simulink model "six_plus_six_AcmsteeringV09_main_2lflm"  (R2014a)
settings: Solver=FixedStepDiscrete  StartTime=0.0  StopTime=10.0  FixedStep=0.0005  RelTol=1e-3
InitFcn:
  | Veh_Par_wxt
undefined symbols (not defined in the file or in its folder): acc_spdctl, ag_thr, B, bra_em, bra_pre_gz2, bra_pre_gz34, bra_pre_yd, brakepre_dem_data, brakeTrq_dem_data, bratrq_max, ecucoder_acal, eff_tran, ESP_switch, G, guzhang_lf, guzhang_lm, guzhang_lr, guzhang_rf, guzhang_rm, guzhang_rr, kd1, kd2, ki1, ki2, kp1, kp2, L, myFIS, premax, Radius, RC_switch, s_opt_yi, s_opt_zhuan, s_opt_zhuan_add, s_opt_zhuan_table, spd_map_mot, spd_spdctl, speed_thr_park, TCS_switch, tras_ratio, trq_map_mot, trqmax_yd, trqmax_zx, trqmaxneg, v_gain, v_table, v_thr_park, zhidong_bianmazhi, zhidong_down, zhidong_up, zhidong_youmen, zhuanxiang_bianmazhi, zhuanxiang_down, zhuanxiang_up, zhuanxiang_youmen
libraries: simulink x980, ec5744lib x59, fuzblock x2
(part 8 of 25)

== system six_plus_six_AcmsteeringV09_main_2lflm/Data_input/MCU0_1/MCU0 ==
  input : Inport
  Enable : EnablePort
  Demux : Demux  Outputs=8
  MCU0_ControlMode_Ad : Sum
  MCU0_ControlMode_Convert : DataTypeConversion  OutDataTypeStr=uint32
  MCU0_ControlMode_F : Gain
  MCU0_ControlMode_L : simulink/Logic and Bit Operations/Bitwise Operator  logicop=AND  UseBitMask=on  BitMask=4  BitMaskRealWorld=Stored Integer
  MCU0_ControlMode_O : Constant  Value=0  OutDataTypeStr=single
  MCU0_ControlMode_S : ArithShift  BitShiftNumber=2
  MCU0_ControlMode_Sub : Subsystem
  MCU0_ControlMode_sat : Saturate  UpperLimit=1  LowerLimit=0
  MCU0_ControlModecv : DataTypeConversion
  MCU0_EmergShutDown_Ad : Sum
  MCU0_EmergShutDown_Convert : DataTypeConversion  OutDataTypeStr=uint32
  MCU0_EmergShutDown_F : Gain
  MCU0_EmergShutDown_L : simulink/Logic and Bit Operations/Bitwise Operator  logicop=AND  UseBitMask=on  BitMask=128  BitMaskRealWorld=Stored Integer
  MCU0_EmergShutDown_O : Constant  Value=0  OutDataTypeStr=single
  MCU0_EmergShutDown_S : ArithShift  BitShiftNumber=7
  MCU0_EmergShutDown_Sub : Subsystem
  MCU0_EmergShutDown_sat : Saturate  UpperLimit=1  LowerLimit=0
  MCU0_EmergShutDowncv : DataTypeConversion
  MCU0_GearStatus_Ad : Sum
  MCU0_GearStatus_Convert : DataTypeConversion  OutDataTypeStr=uint32
  MCU0_GearStatus_F : Gain
  MCU0_GearStatus_L : simulink/Logic and Bit Operations/Bitwise Operator  logicop=AND  UseBitMask=on  BitMask=24  BitMaskRealWorld=Stored Integer
  MCU0_GearStatus_O : Constant  Value=0  OutDataTypeStr=single
  MCU0_GearStatus_S : ArithShift  BitShiftNumber=3
  MCU0_GearStatus_Sub : Subsystem
  MCU0_GearStatus_sat : Saturate  UpperLimit=3  LowerLimit=0
  MCU0_GearStatuscv : DataTypeConversion
  MCU0_HighVol_Ad : Sum
  MCU0_HighVol_Convert : DataTypeConversion  OutDataTypeStr=uint32
  MCU0_HighVol_F : Gain
  MCU0_HighVol_L : simulink/Logic and Bit Operations/Bitwise Operator  logicop=AND  UseBitMask=on  BitMask=32  BitMaskRealWorld=Stored Integer
  MCU0_HighVol_O : Constant  Value=0  OutDataTypeStr=single
  MCU0_HighVol_S : ArithShift  BitShiftNumber=5
  MCU0_HighVol_Sub : Subsystem
  MCU0_HighVol_sat : Saturate  UpperLimit=1  LowerLimit=0
  MCU0_HighVolcv : DataTypeConversion
  MCU0_LiftCnt_Ad : Sum
  MCU0_LiftCnt_Convert : DataTypeConversion  OutDataTypeStr=uint32
  MCU0_LiftCnt_F : Gain
  MCU0_LiftCnt_L : simulink/Logic and Bit Operations/Bitwise Operator  logicop=AND  UseBitMask=on  BitMask=255  BitMaskRealWorld=Stored Integer
  MCU0_LiftCnt_O : Constant  Value=0  OutDataTypeStr=single
  MCU0_LiftCnt_S : ArithShift
  MCU0_LiftCnt_Sub : Subsystem
  MCU0_LiftCnt_sat : Saturate  UpperLimit=255  LowerLimit=0
  MCU0_LiftCntcv : DataTypeConversion
  MCU0_ShutDowAllow_Ad : Sum
  MCU0_ShutDowAllow_Convert : DataTypeConversion  OutDataTypeStr=uint32
  MCU0_ShutDowAllow_F : Gain
  MCU0_ShutDowAllow_L : simulink/Logic and Bit Operations/Bitwise Operator  logicop=AND  UseBitMask=on  BitMask=64  BitMaskRealWorld=Stored Integer
  MCU0_ShutDowAllow_O : Constant  Value=0  OutDataTypeStr=single
  MCU0_ShutDowAllow_S : ArithShift  BitShiftNumber=6
  MCU0_ShutDowAllow_Sub : Subsystem
  MCU0_ShutDowAllow_sat : Saturate  UpperLimit=1  LowerLimit=0
  MCU0_ShutDowAllowcv : DataTypeConversion
  MCU0_SpeedFdk_Ad : Sum
  MCU0_SpeedFdk_Convert : DataTypeConversion  OutDataTypeStr=uint32
  MCU0_SpeedFdk_F : Gain
  MCU0_SpeedFdk_L : simulink/Logic and Bit Operations/Bitwise Operator  logicop=AND  UseBitMask=on  BitMask=65535  BitMaskRealWorld=Stored Integer
  MCU0_SpeedFdk_O : Constant  Value=-10000  OutDataTypeStr=single
  MCU0_SpeedFdk_S : ArithShift
  MCU0_SpeedFdk_Sub : Subsystem
  MCU0_SpeedFdk_sat : Saturate  UpperLimit=10000  LowerLimit=-10000
  MCU0_SpeedFdkcv : DataTypeConversion
  MCU0_SpeedFdkinput2_Ad : Sum
  MCU0_SpeedFdkinput2_C : Constant  Value=256
  MCU0_SpeedFdkinput2_P : Product
  MCU0_TorqueFdk_Ad : Sum
  MCU0_TorqueFdk_Convert : DataTypeConversion  OutDataTypeStr=uint32
  MCU0_TorqueFdk_F : Gain  Gain=0.1
  MCU0_TorqueFdk_L : simulink/Logic and Bit Operations/Bitwise Operator  logicop=AND  UseBitMask=on  BitMask=65535  BitMaskRealWorld=Stored Integer
  MCU0_TorqueFdk_O : Constant  Value=-1000  OutDataTypeStr=single
  MCU0_TorqueFdk_S : ArithShift
  MCU0_TorqueFdk_Sub : Subsystem
  MCU0_TorqueFdk_sat : Saturate  UpperLimit=1000  LowerLimit=-1000
  MCU0_TorqueFdkcv : DataTypeConversion
  MCU0_TorqueFdkinput4_Ad : Sum
  MCU0_TorqueFdkinput4_C : Constant  Value=256
  MCU0_TorqueFdkinput4_P : Product
  MCU0_TorqueMax_Ad : Sum
  MCU0_TorqueMax_Convert : DataTypeConversion  OutDataTypeStr=uint32
  MCU0_TorqueMax_F : Gain  Gain=0.1
  MCU0_TorqueMax_L : simulink/Logic and Bit Operations/Bitwise Operator  logicop=AND  UseBitMask=on  BitMask=65535  BitMaskRealWorld=Stored Integer
  MCU0_TorqueMax_O : Constant  Value=-1000  OutDataTypeStr=single
  MCU0_TorqueMax_S : ArithShift
  MCU0_TorqueMax_Sub : Subsystem
  MCU0_TorqueMax_sat : Saturate  UpperLimit=1000  LowerLimit=-1000
  MCU0_TorqueMaxcv : DataTypeConversion
  MCU0_TorqueMaxinput6_Ad : Sum
  MCU0_TorqueMaxinput6_C : Constant  Value=256
  MCU0_TorqueMaxinput6_P : Product
  MCU0_WorkStatus_Ad : Sum
  MCU0_WorkStatus_Convert : DataTypeConversion  OutDataTypeStr=uint32
  MCU0_WorkStatus_F : Gain
  MCU0_WorkStatus_L : simulink/Logic and Bit Operations/Bitwise Operator  logicop=AND  UseBitMask=on  BitMask=3  BitMaskRealWorld=Stored Integer
  MCU0_WorkStatus_O : Constant  Value=0  OutDataTypeStr=single
  MCU0_WorkStatus_S : ArithShift
  MCU0_WorkStatus_Sub : Subsystem
  MCU0_WorkStatus_sat : Saturate  UpperLimit=3  LowerLimit=0
  MCU0_WorkStatuscv : DataTypeConversion
  MCU0_TorqueMax_Out : Outport
  MCU0_EmergShutDown_Out : Outport  Port=2
  MCU0_ShutDowAllow_Out : Outport  Port=3
  MCU0_HighVol_Out : Outport  Port=4
  MCU0_LiftCnt_Out : Outport  Port=5
  MCU0_TorqueFdk_Out : Outport  Port=6
  MCU0_SpeedFdk_Out : Outport  Port=7
  MCU0_GearStatus_Out : Outport  Port=8
  MCU0_ControlMode_Out : Outport  Port=9
  MCU0_WorkStatus_Out : Outport  Port=10
  wires:
  MCU0_TorqueMax_F/1 -> MCU0_TorqueMax_Ad/1
  MCU0_TorqueMax_O/1 -> MCU0_TorqueMax_Ad/2
  MCU0_TorqueMax_Ad/1 -> MCU0_TorqueMax_sat/1
  MCU0_TorqueMax_sat/1 -> MCU0_TorqueMax_Out/1
  Demux/6 -> MCU0_TorqueMaxinput6_P/1
  MCU0_TorqueMaxinput6_C/1 -> MCU0_TorqueMaxinput6_P/2
  MCU0_TorqueMaxinput6_P/1 -> MCU0_TorqueMaxinput6_Ad/1
  Demux/7 -> MCU0_TorqueMaxinput6_Ad/2
  MCU0_TorqueMaxinput6_Ad/1 -> MCU0_TorqueMax_Sub/1(In1)
  MCU0_TorqueMax_Sub/1(Out1) -> MCU0_TorqueMax_Convert/1
  MCU0_TorqueMax_Convert/1 -> MCU0_TorqueMax_L/1
  MCU0_TorqueMax_L/1 -> MCU0_TorqueMax_S/1
  MCU0_TorqueMax_S/1 -> MCU0_TorqueMaxcv/1
  MCU0_TorqueMaxcv/1 -> MCU0_TorqueMax_F/1
  MCU0_EmergShutDown_F/1 -> MCU0_EmergShutDown_Ad/1
  MCU0_EmergShutDown_O/1 -> MCU0_EmergShutDown_Ad/2
  MCU0_EmergShutDown_Ad/1 -> MCU0_EmergShutDown_sat/1
  MCU0_EmergShutDown_sat/1 -> MCU0_EmergShutDown_Out/1
  Demux/1 -> MCU0_ControlMode_Sub/1(In1), MCU0_WorkStatus_Sub/1(In1), MCU0_GearStatus_Sub/1(In1), MCU0_HighVol_Sub/1(In1), MCU0_ShutDowAllow_Sub/1(In1), MCU0_EmergShutDown_Sub/1(In1)
  MCU0_EmergShutDown_Sub/1(Out1) -> MCU0_EmergShutDown_Convert/1
  MCU0_EmergShutDown_Convert/1 -> MCU0_EmergShutDown_L/1
  MCU0_EmergShutDown_L/1 -> MCU0_EmergShutDown_S/1
  MCU0_EmergShutDown_S/1 -> MCU0_EmergShutDowncv/1
  MCU0_EmergShutDowncv/1 -> MCU0_EmergShutDown_F/1
  MCU0_ShutDowAllow_F/1 -> MCU0_ShutDowAllow_Ad/1
  MCU0_ShutDowAllow_O/1 -> MCU0_ShutDowAllow_Ad/2
  MCU0_ShutDowAllow_Ad/1 -> MCU0_ShutDowAllow_sat/1
  MCU0_ShutDowAllow_sat/1 -> MCU0_ShutDowAllow_Out/1
  MCU0_ShutDowAllow_Sub/1(Out1) -> MCU0_ShutDowAllow_Convert/1
  MCU0_ShutDowAllow_Convert/1 -> MCU0_ShutDowAllow_L/1
  MCU0_ShutDowAllow_L/1 -> MCU0_ShutDowAllow_S/1
  MCU0_ShutDowAllow_S/1 -> MCU0_ShutDowAllowcv/1
  MCU0_ShutDowAllowcv/1 -> MCU0_ShutDowAllow_F/1
  MCU0_HighVol_F/1 -> MCU0_HighVol_Ad/1
  MCU0_HighVol_O/1 -> MCU0_HighVol_Ad/2
  MCU0_HighVol_Ad/1 -> MCU0_HighVol_sat/1
  MCU0_HighVol_sat/1 -> MCU0_HighVol_Out/1
  MCU0_HighVol_Sub/1(Out1) -> MCU0_HighVol_Convert/1
  MCU0_HighVol_Convert/1 -> MCU0_HighVol_L/1
  MCU0_HighVol_L/1 -> MCU0_HighVol_S/1
  MCU0_HighVol_S/1 -> MCU0_HighVolcv/1
  MCU0_HighVolcv/1 -> MCU0_HighVol_F/1
  MCU0_LiftCnt_F/1 -> MCU0_LiftCnt_Ad/1
  MCU0_LiftCnt_O/1 -> MCU0_LiftCnt_Ad/2
  MCU0_LiftCnt_Ad/1 -> MCU0_LiftCnt_sat/1
  MCU0_LiftCnt_sat/1 -> MCU0_LiftCnt_Out/1
  Demux/8 -> MCU0_LiftCnt_Sub/1(In1)
  MCU0_LiftCnt_Sub/1(Out1) -> MCU0_LiftCnt_Convert/1
  MCU0_LiftCnt_Convert/1 -> MCU0_LiftCnt_L/1
  MCU0_LiftCnt_L/1 -> MCU0_LiftCnt_S/1
  MCU0_LiftCnt_S/1 -> MCU0_LiftCntcv/1
  MCU0_LiftCntcv/1 -> MCU0_LiftCnt_F/1
  MCU0_TorqueFdk_F/1 -> MCU0_TorqueFdk_Ad/1
  MCU0_TorqueFdk_O/1 -> MCU0_TorqueFdk_Ad/2
  MCU0_TorqueFdk_Ad/1 -> MCU0_TorqueFdk_sat/1
  MCU0_TorqueFdk_sat/1 -> MCU0_TorqueFdk_Out/1
  Demux/4 -> MCU0_TorqueFdkinput4_P/1
  MCU0_TorqueFdkinput4_C/1 -> MCU0_TorqueFdkinput4_P/2
  MCU0_TorqueFdkinput4_P/1 -> MCU0_TorqueFdkinput4_Ad/1
  Demux/5 -> MCU0_TorqueFdkinput4_Ad/2
  MCU0_TorqueFdkinput4_Ad/1 -> MCU0_TorqueFdk_Sub/1(In1)
  MCU0_TorqueFdk_Sub/1(Out1) -> MCU0_TorqueFdk_Convert/1
  MCU0_TorqueFdk_Convert/1 -> MCU0_TorqueFdk_L/1
  MCU0_TorqueFdk_L/1 -> MCU0_TorqueFdk_S/1
  MCU0_TorqueFdk_S/1 -> MCU0_TorqueFdkcv/1
  MCU0_TorqueFdkcv/1 -> MCU0_TorqueFdk_F/1
  MCU0_SpeedFdk_F/1 -> MCU0_SpeedFdk_Ad/1
  MCU0_SpeedFdk_O/1 -> MCU0_SpeedFdk_Ad/2
  MCU0_SpeedFdk_Ad/1 -> MCU0_SpeedFdk_sat/1
  MCU0_SpeedFdk_sat/1 -> MCU0_SpeedFdk_Out/1
  Demux/2 -> MCU0_SpeedFdkinput2_P/1
  MCU0_SpeedFdkinput2_C/1 -> MCU0_SpeedFdkinput2_P/2
  MCU0_SpeedFdkinput2_P/1 -> MCU0_SpeedFdkinput2_Ad/1
  Demux/3 -> MCU0_SpeedFdkinput2_Ad/2
  MCU0_SpeedFdkinput2_Ad/1 -> MCU0_SpeedFdk_Sub/1(In1)
  MCU0_SpeedFdk_Sub/1(Out1) -> MCU0_SpeedFdk_Convert/1
  MCU0_SpeedFdk_Convert/1 -> MCU0_SpeedFdk_L/1
  MCU0_SpeedFdk_L/1 -> MCU0_SpeedFdk_S/1
  MCU0_SpeedFdk_S/1 -> MCU0_SpeedFdkcv/1
  MCU0_SpeedFdkcv/1 -> MCU0_SpeedFdk_F/1
  MCU0_GearStatus_F/1 -> MCU0_GearStatus_Ad/1
  MCU0_GearStatus_O/1 -> MCU0_GearStatus_Ad/2
  MCU0_GearStatus_Ad/1 -> MCU0_GearStatus_sat/1
  MCU0_GearStatus_sat/1 -> MCU0_GearStatus_Out/1
  MCU0_GearStatus_Sub/1(Out1) -> MCU0_GearStatus_Convert/1
  MCU0_GearStatus_Convert/1 -> MCU0_GearStatus_L/1
  MCU0_GearStatus_L/1 -> MCU0_GearStatus_S/1
  MCU0_GearStatus_S/1 -> MCU0_GearStatuscv/1
  MCU0_GearStatuscv/1 -> MCU0_GearStatus_F/1
  MCU0_ControlMode_F/1 -> MCU0_ControlMode_Ad/1
  MCU0_ControlMode_O/1 -> MCU0_ControlMode_Ad/2
  MCU0_ControlMode_Ad/1 -> MCU0_ControlMode_sat/1
  MCU0_ControlMode_sat/1 -> MCU0_ControlMode_Out/1
  MCU0_ControlMode_Sub/1(Out1) -> MCU0_ControlMode_Convert/1
  MCU0_ControlMode_Convert/1 -> MCU0_ControlMode_L/1
  MCU0_ControlMode_L/1 -> MCU0_ControlMode_S/1
  MCU0_ControlMode_S/1 -> MCU0_ControlModecv/1
  MCU0_ControlModecv/1 -> MCU0_ControlMode_F/1
  MCU0_WorkStatus_F/1 -> MCU0_WorkStatus_Ad/1
  MCU0_WorkStatus_O/1 -> MCU0_WorkStatus_Ad/2
  MCU0_WorkStatus_Ad/1 -> MCU0_WorkStatus_sat/1
  MCU0_WorkStatus_sat/1 -> MCU0_WorkStatus_Out/1
  MCU0_WorkStatus_Sub/1(Out1) -> MCU0_WorkStatus_Convert/1
  MCU0_WorkStatus_Convert/1 -> MCU0_WorkStatus_L/1
  MCU0_WorkStatus_L/1 -> MCU0_WorkStatus_S/1
  MCU0_WorkStatus_S/1 -> MCU0_WorkStatuscv/1
  MCU0_WorkStatuscv/1 -> MCU0_WorkStatus_F/1
  input/1 -> Demux/1

== system six_plus_six_AcmsteeringV09_main_2lflm/Data_input/MCU0_2/MCU0 ==
  input : Inport
  Enable : EnablePort
  Demux : Demux  Outputs=8
  MCU0_ControlMode_Ad : Sum
  MCU0_ControlMode_Convert : DataTypeConversion  OutDataTypeStr=uint32
  MCU0_ControlMode_F : Gain
  MCU0_ControlMode_L : simulink/Logic and Bit Operations/Bitwise Operator  logicop=AND  UseBitMask=on  BitMask=4  BitMaskRealWorld=Stored Integer
  MCU0_ControlMode_O : Constant  Value=0  OutDataTypeStr=single
  MCU0_ControlMode_S : ArithShift  BitShiftNumber=2
  MCU0_ControlMode_Sub : Subsystem
  MCU0_ControlMode_sat : Saturate  UpperLimit=1  LowerLimit=0
  MCU0_ControlModecv : DataTypeConversion
  MCU0_EmergShutDown_Ad : Sum
  MCU0_EmergShutDown_Convert : DataTypeConversion  OutDataTypeStr=uint32
  MCU0_EmergShutDown_F : Gain
  MCU0_EmergShutDown_L : simulink/Logic and Bit Operations/Bitwise Operator  logicop=AND  UseBitMask=on  BitMask=128  BitMaskRealWorld=Stored Integer
  MCU0_EmergShutDown_O : Constant  Value=0  OutDataTypeStr=single
  MCU0_EmergShutDown_S : ArithShift  BitShiftNumber=7
  MCU0_EmergShutDown_Sub : Subsystem
  MCU0_EmergShutDown_sat : Saturate  UpperLimit=1  LowerLimit=0
  MCU0_EmergShutDowncv : DataTypeConversion
  MCU0_GearStatus_Ad : Sum
  MCU0_GearStatus_Convert : DataTypeConversion  OutDataTypeStr=uint32
  MCU0_GearStatus_F : Gain
  MCU0_GearStatus_L : simulink/Logic and Bit Operations/Bitwise Operator  logicop=AND  UseBitMask=on  BitMask=24  BitMaskRealWorld=Stored Integer
  MCU0_GearStatus_O : Constant  Value=0  OutDataTypeStr=single
  MCU0_GearStatus_S : ArithShift  BitShiftNumber=3
  MCU0_GearStatus_Sub : Subsystem
  MCU0_GearStatus_sat : Saturate  UpperLimit=3  LowerLimit=0
  MCU0_GearStatuscv : DataTypeConversion
  MCU0_HighVol_Ad : Sum
  MCU0_HighVol_Convert : DataTypeConversion  OutDataTypeStr=uint32
  MCU0_HighVol_F : Gain
  MCU0_HighVol_L : simulink/Logic and Bit Operations/Bitwise Operator  logicop=AND  UseBitMask=on  BitMask=32  BitMaskRealWorld=Stored Integer
  MCU0_HighVol_O : Constant  Value=0  OutDataTypeStr=single
  MCU0_HighVol_S : ArithShift  BitShiftNumber=5
  MCU0_HighVol_Sub : Subsystem
  MCU0_HighVol_sat : Saturate  UpperLimit=1  LowerLimit=0
  MCU0_HighVolcv : DataTypeConversion
  MCU0_LiftCnt_Ad : Sum
  MCU0_LiftCnt_Convert : DataTypeConversion  OutDataTypeStr=uint32
  MCU0_LiftCnt_F : Gain
  MCU0_LiftCnt_L : simulink/Logic and Bit Operations/Bitwise Operator  logicop=AND  UseBitMask=on  BitMask=255  BitMaskRealWorld=Stored Integer
  MCU0_LiftCnt_O : Constant  Value=0  OutDataTypeStr=single
  MCU0_LiftCnt_S : ArithShift
  MCU0_LiftCnt_Sub : Subsystem
  MCU0_LiftCnt_sat : Saturate  UpperLimit=255  LowerLimit=0
  MCU0_LiftCntcv : DataTypeConversion
  MCU0_ShutDowAllow_Ad : Sum
  MCU0_ShutDowAllow_Convert : DataTypeConversion  OutDataTypeStr=uint32
  MCU0_ShutDowAllow_F : Gain
  MCU0_ShutDowAllow_L : simulink/Logic and Bit Operations/Bitwise Operator  logicop=AND  UseBitMask=on  BitMask=64  BitMaskRealWorld=Stored Integer
  MCU0_ShutDowAllow_O : Constant  Value=0  OutDataTypeStr=single
  MCU0_ShutDowAllow_S : ArithShift  BitShiftNumber=6
  MCU0_ShutDowAllow_Sub : Subsystem
  MCU0_ShutDowAllow_sat : Saturate  UpperLimit=1  LowerLimit=0
  MCU0_ShutDowAllowcv : DataTypeConversion
  MCU0_SpeedFdk_Ad : Sum
  MCU0_SpeedFdk_Convert : DataTypeConversion  OutDataTypeStr=uint32
  MCU0_SpeedFdk_F : Gain
  MCU0_SpeedFdk_L : simulink/Logic and Bit Operations/Bitwise Operator  logicop=AND  UseBitMask=on  BitMask=65535  BitMaskRealWorld=Stored Integer
  MCU0_SpeedFdk_O : Constant  Value=-10000  OutDataTypeStr=single
  MCU0_SpeedFdk_S : ArithShift
  MCU0_SpeedFdk_Sub : Subsystem
  MCU0_SpeedFdk_sat : Saturate  UpperLimit=10000  LowerLimit=-10000
  MCU0_SpeedFdkcv : DataTypeConversion
  MCU0_SpeedFdkinput2_Ad : Sum
  MCU0_SpeedFdkinput2_C : Constant  Value=256
  MCU0_SpeedFdkinput2_P : Product
  MCU0_TorqueFdk_Ad : Sum
  MCU0_TorqueFdk_Convert : DataTypeConversion  OutDataTypeStr=uint32
  MCU0_TorqueFdk_F : Gain  Gain=0.1
  MCU0_TorqueFdk_L : simulink/Logic and Bit Operations/Bitwise Operator  logicop=AND  UseBitMask=on  BitMask=65535  BitMaskRealWorld=Stored Integer
  MCU0_TorqueFdk_O : Constant  Value=-1000  OutDataTypeStr=single
  MCU0_TorqueFdk_S : ArithShift
  MCU0_TorqueFdk_Sub : Subsystem
  MCU0_TorqueFdk_sat : Saturate  UpperLimit=1000  LowerLimit=-1000
  MCU0_TorqueFdkcv : DataTypeConversion
  MCU0_TorqueFdkinput4_Ad : Sum
  MCU0_TorqueFdkinput4_C : Constant  Value=256
  MCU0_TorqueFdkinput4_P : Product
  MCU0_TorqueMax_Ad : Sum
  MCU0_TorqueMax_Convert : DataTypeConversion  OutDataTypeStr=uint32
  MCU0_TorqueMax_F : Gain  Gain=0.1
  MCU0_TorqueMax_L : simulink/Logic and Bit Operations/Bitwise Operator  logicop=AND  UseBitMask=on  BitMask=65535  BitMaskRealWorld=Stored Integer
  MCU0_TorqueMax_O : Constant  Value=-1000  OutDataTypeStr=single
  MCU0_TorqueMax_S : ArithShift
  MCU0_TorqueMax_Sub : Subsystem
  MCU0_TorqueMax_sat : Saturate  UpperLimit=1000  LowerLimit=-1000
  MCU0_TorqueMaxcv : DataTypeConversion
  MCU0_TorqueMaxinput6_Ad : Sum
  MCU0_TorqueMaxinput6_C : Constant  Value=256
  MCU0_TorqueMaxinput6_P : Product
  MCU0_WorkStatus_Ad : Sum
  MCU0_WorkStatus_Convert : DataTypeConversion  OutDataTypeStr=uint32
  MCU0_WorkStatus_F : Gain
  MCU0_WorkStatus_L : simulink/Logic and Bit Operations/Bitwise Operator  logicop=AND  UseBitMask=on  BitMask=3  BitMaskRealWorld=Stored Integer
  MCU0_WorkStatus_O : Constant  Value=0  OutDataTypeStr=single
  MCU0_WorkStatus_S : ArithShift
  MCU0_WorkStatus_Sub : Subsystem
  MCU0_WorkStatus_sat : Saturate  UpperLimit=3  LowerLimit=0
  MCU0_WorkStatuscv : DataTypeConversion
  MCU0_TorqueMax_Out : Outport
  MCU0_EmergShutDown_Out : Outport  Port=2
  MCU0_ShutDowAllow_Out : Outport  Port=3
  MCU0_HighVol_Out : Outport  Port=4
  MCU0_LiftCnt_Out : Outport  Port=5
  MCU0_TorqueFdk_Out : Outport  Port=6
  MCU0_SpeedFdk_Out : Outport  Port=7
  MCU0_GearStatus_Out : Outport  Port=8
  MCU0_ControlMode_Out : Outport  Port=9
  MCU0_WorkStatus_Out : Outport  Port=10
  wires:
  MCU0_TorqueMax_F/1 -> MCU0_TorqueMax_Ad/1
  MCU0_TorqueMax_O/1 -> MCU0_TorqueMax_Ad/2
  MCU0_TorqueMax_Ad/1 -> MCU0_TorqueMax_sat/1
  MCU0_TorqueMax_sat/1 -> MCU0_TorqueMax_Out/1
  Demux/6 -> MCU0_TorqueMaxinput6_P/1
  MCU0_TorqueMaxinput6_C/1 -> MCU0_TorqueMaxinput6_P/2
  MCU0_TorqueMaxinput6_P/1 -> MCU0_TorqueMaxinput6_Ad/1
  Demux/7 -> MCU0_TorqueMaxinput6_Ad/2
  MCU0_TorqueMaxinput6_Ad/1 -> MCU0_TorqueMax_Sub/1(In1)
  MCU0_TorqueMax_Sub/1(Out1) -> MCU0_TorqueMax_Convert/1
  MCU0_TorqueMax_Convert/1 -> MCU0_TorqueMax_L/1
  MCU0_TorqueMax_L/1 -> MCU0_TorqueMax_S/1
  MCU0_TorqueMax_S/1 -> MCU0_TorqueMaxcv/1
  MCU0_TorqueMaxcv/1 -> MCU0_TorqueMax_F/1
  MCU0_EmergShutDown_F/1 -> MCU0_EmergShutDown_Ad/1
  MCU0_EmergShutDown_O/1 -> MCU0_EmergShutDown_Ad/2
  MCU0_EmergShutDown_Ad/1 -> MCU0_EmergShutDown_sat/1
  MCU0_EmergShutDown_sat/1 -> MCU0_EmergShutDown_Out/1
  Demux/1 -> MCU0_ControlMode_Sub/1(In1), MCU0_WorkStatus_Sub/1(In1), MCU0_GearStatus_Sub/1(In1), MCU0_HighVol_Sub/1(In1), MCU0_ShutDowAllow_Sub/1(In1), MCU0_EmergShutDown_Sub/1(In1)
  MCU0_EmergShutDown_Sub/1(Out1) -> MCU0_EmergShutDown_Convert/1
  MCU0_EmergShutDown_Convert/1 -> MCU0_EmergShutDown_L/1
  MCU0_EmergShutDown_L/1 -> MCU0_EmergShutDown_S/1
  MCU0_EmergShutDown_S/1 -> MCU0_EmergShutDowncv/1
  MCU0_EmergShutDowncv/1 -> MCU0_EmergShutDown_F/1
  MCU0_ShutDowAllow_F/1 -> MCU0_ShutDowAllow_Ad/1
  MCU0_ShutDowAllow_O/1 -> MCU0_ShutDowAllow_Ad/2
  MCU0_ShutDowAllow_Ad/1 -> MCU0_ShutDowAllow_sat/1
  MCU0_ShutDowAllow_sat/1 -> MCU0_ShutDowAllow_Out/1
  MCU0_ShutDowAllow_Sub/1(Out1) -> MCU0_ShutDowAllow_Convert/1
  MCU0_ShutDowAllow_Convert/1 -> MCU0_ShutDowAllow_L/1
  MCU0_ShutDowAllow_L/1 -> MCU0_ShutDowAllow_S/1
  MCU0_ShutDowAllow_S/1 -> MCU0_ShutDowAllowcv/1
  MCU0_ShutDowAllowcv/1 -> MCU0_ShutDowAllow_F/1
  MCU0_HighVol_F/1 -> MCU0_HighVol_Ad/1
  MCU0_HighVol_O/1 -> MCU0_HighVol_Ad/2
  MCU0_HighVol_Ad/1 -> MCU0_HighVol_sat/1
  MCU0_HighVol_sat/1 -> MCU0_HighVol_Out/1
  MCU0_HighVol_Sub/1(Out1) -> MCU0_HighVol_Convert/1
  MCU0_HighVol_Convert/1 -> MCU0_HighVol_L/1
  MCU0_HighVol_L/1 -> MCU0_HighVol_S/1
  MCU0_HighVol_S/1 -> MCU0_HighVolcv/1
  MCU0_HighVolcv/1 -> MCU0_HighVol_F/1
  MCU0_LiftCnt_F/1 -> MCU0_LiftCnt_Ad/1
  MCU0_LiftCnt_O/1 -> MCU0_LiftCnt_Ad/2
  MCU0_LiftCnt_Ad/1 -> MCU0_LiftCnt_sat/1
  MCU0_LiftCnt_sat/1 -> MCU0_LiftCnt_Out/1
  Demux/8 -> MCU0_LiftCnt_Sub/1(In1)
  MCU0_LiftCnt_Sub/1(Out1) -> MCU0_LiftCnt_Convert/1
  MCU0_LiftCnt_Convert/1 -> MCU0_LiftCnt_L/1
  MCU0_LiftCnt_L/1 -> MCU0_LiftCnt_S/1
  MCU0_LiftCnt_S/1 -> MCU0_LiftCntcv/1
  MCU0_LiftCntcv/1 -> MCU0_LiftCnt_F/1
  MCU0_TorqueFdk_F/1 -> MCU0_TorqueFdk_Ad/1
  MCU0_TorqueFdk_O/1 -> MCU0_TorqueFdk_Ad/2
  MCU0_TorqueFdk_Ad/1 -> MCU0_TorqueFdk_sat/1
  MCU0_TorqueFdk_sat/1 -> MCU0_TorqueFdk_Out/1
  Demux/4 -> MCU0_TorqueFdkinput4_P/1
  MCU0_TorqueFdkinput4_C/1 -> MCU0_TorqueFdkinput4_P/2
  MCU0_TorqueFdkinput4_P/1 -> MCU0_TorqueFdkinput4_Ad/1
  Demux/5 -> MCU0_TorqueFdkinput4_Ad/2
  MCU0_TorqueFdkinput4_Ad/1 -> MCU0_TorqueFdk_Sub/1(In1)
  MCU0_TorqueFdk_Sub/1(Out1) -> MCU0_TorqueFdk_Convert/1
  MCU0_TorqueFdk_Convert/1 -> MCU0_TorqueFdk_L/1
  MCU0_TorqueFdk_L/1 -> MCU0_TorqueFdk_S/1
  MCU0_TorqueFdk_S/1 -> MCU0_TorqueFdkcv/1
  MCU0_TorqueFdkcv/1 -> MCU0_TorqueFdk_F/1
  MCU0_SpeedFdk_F/1 -> MCU0_SpeedFdk_Ad/1
  MCU0_SpeedFdk_O/1 -> MCU0_SpeedFdk_Ad/2
  MCU0_SpeedFdk_Ad/1 -> MCU0_SpeedFdk_sat/1
  MCU0_SpeedFdk_sat/1 -> MCU0_SpeedFdk_Out/1
  Demux/2 -> MCU0_SpeedFdkinput2_P/1
  MCU0_SpeedFdkinput2_C/1 -> MCU0_SpeedFdkinput2_P/2
  MCU0_SpeedFdkinput2_P/1 -> MCU0_SpeedFdkinput2_Ad/1
  Demux/3 -> MCU0_SpeedFdkinput2_Ad/2
  MCU0_SpeedFdkinput2_Ad/1 -> MCU0_SpeedFdk_Sub/1(In1)
  MCU0_SpeedFdk_Sub/1(Out1) -> MCU0_SpeedFdk_Convert/1
  MCU0_SpeedFdk_Convert/1 -> MCU0_SpeedFdk_L/1
  MCU0_SpeedFdk_L/1 -> MCU0_SpeedFdk_S/1
  MCU0_SpeedFdk_S/1 -> MCU0_SpeedFdkcv/1
  MCU0_SpeedFdkcv/1 -> MCU0_SpeedFdk_F/1
  MCU0_GearStatus_F/1 -> MCU0_GearStatus_Ad/1
  MCU0_GearStatus_O/1 -> MCU0_GearStatus_Ad/2
  MCU0_GearStatus_Ad/1 -> MCU0_GearStatus_sat/1
  MCU0_GearStatus_sat/1 -> MCU0_GearStatus_Out/1
  MCU0_GearStatus_Sub/1(Out1) -> MCU0_GearStatus_Convert/1
  MCU0_GearStatus_Convert/1 -> MCU0_GearStatus_L/1
  MCU0_GearStatus_L/1 -> MCU0_GearStatus_S/1
  MCU0_GearStatus_S/1 -> MCU0_GearStatuscv/1
  MCU0_GearStatuscv/1 -> MCU0_GearStatus_F/1
  MCU0_ControlMode_F/1 -> MCU0_ControlMode_Ad/1
  MCU0_ControlMode_O/1 -> MCU0_ControlMode_Ad/2
  MCU0_ControlMode_Ad/1 -> MCU0_ControlMode_sat/1
  MCU0_ControlMode_sat/1 -> MCU0_ControlMode_Out/1
  MCU0_ControlMode_Sub/1(Out1) -> MCU0_ControlMode_Convert/1
  MCU0_ControlMode_Convert/1 -> MCU0_ControlMode_L/1
  MCU0_ControlMode_L/1 -> MCU0_ControlMode_S/1
  MCU0_ControlMode_S/1 -> MCU0_ControlModecv/1
  MCU0_ControlModecv/1 -> MCU0_ControlMode_F/1
  MCU0_WorkStatus_F/1 -> MCU0_WorkStatus_Ad/1
  MCU0_WorkStatus_O/1 -> MCU0_WorkStatus_Ad/2
  MCU0_WorkStatus_Ad/1 -> MCU0_WorkStatus_sat/1
  MCU0_WorkStatus_sat/1 -> MCU0_WorkStatus_Out/1
  MCU0_WorkStatus_Sub/1(Out1) -> MCU0_WorkStatus_Convert/1
  MCU0_WorkStatus_Convert/1 -> MCU0_WorkStatus_L/1
  MCU0_WorkStatus_L/1 -> MCU0_WorkStatus_S/1
  MCU0_WorkStatus_S/1 -> MCU0_WorkStatuscv/1
  MCU0_WorkStatuscv/1 -> MCU0_WorkStatus_F/1
  input/1 -> Demux/1

== system six_plus_six_AcmsteeringV09_main_2lflm/Data_input/MCU0_3/MCU0 ==
  input : Inport
  Enable : EnablePort
  Demux : Demux  Outputs=8
  MCU0_ControlMode_Ad : Sum
  MCU0_ControlMode_Convert : DataTypeConversion  OutDataTypeStr=uint32
  MCU0_ControlMode_F : Gain
  MCU0_ControlMode_L : simulink/Logic and Bit Operations/Bitwise Operator  logicop=AND  UseBitMask=on  BitMask=4  BitMaskRealWorld=Stored Integer
  MCU0_ControlMode_O : Constant  Value=0  OutDataTypeStr=single
  MCU0_ControlMode_S : ArithShift  BitShiftNumber=2
  MCU0_ControlMode_Sub : Subsystem
  MCU0_ControlMode_sat : Saturate  UpperLimit=1  LowerLimit=0
  MCU0_ControlModecv : DataTypeConversion
  MCU0_EmergShutDown_Ad : Sum
  MCU0_EmergShutDown_Convert : DataTypeConversion  OutDataTypeStr=uint32
  MCU0_EmergShutDown_F : Gain
  MCU0_EmergShutDown_L : simulink/Logic and Bit Operations/Bitwise Operator  logicop=AND  UseBitMask=on  BitMask=128  BitMaskRealWorld=Stored Integer
  MCU0_EmergShutDown_O : Constant  Value=0  OutDataTypeStr=single
  MCU0_EmergShutDown_S : ArithShift  BitShiftNumber=7
  MCU0_EmergShutDown_Sub : Subsystem
  MCU0_EmergShutDown_sat : Saturate  UpperLimit=1  LowerLimit=0
  MCU0_EmergShutDowncv : DataTypeConversion
  MCU0_GearStatus_Ad : Sum
  MCU0_GearStatus_Convert : DataTypeConversion  OutDataTypeStr=uint32
  MCU0_GearStatus_F : Gain
  MCU0_GearStatus_L : simulink/Logic and Bit Operations/Bitwise Operator  logicop=AND  UseBitMask=on  BitMask=24  BitMaskRealWorld=Stored Integer
  MCU0_GearStatus_O : Constant  Value=0  OutDataTypeStr=single
  MCU0_GearStatus_S : ArithShift  BitShiftNumber=3
  MCU0_GearStatus_Sub : Subsystem
  MCU0_GearStatus_sat : Saturate  UpperLimit=3  LowerLimit=0
  MCU0_GearStatuscv : DataTypeConversion
  MCU0_HighVol_Ad : Sum
  MCU0_HighVol_Convert : DataTypeConversion  OutDataTypeStr=uint32
  MCU0_HighVol_F : Gain
  MCU0_HighVol_L : simulink/Logic and Bit Operations/Bitwise Operator  logicop=AND  UseBitMask=on  BitMask=32  BitMaskRealWorld=Stored Integer
  MCU0_HighVol_O : Constant  Value=0  OutDataTypeStr=single
  MCU0_HighVol_S : ArithShift  BitShiftNumber=5
  MCU0_HighVol_Sub : Subsystem
  MCU0_HighVol_sat : Saturate  UpperLimit=1  LowerLimit=0
  MCU0_HighVolcv : DataTypeConversion
  MCU0_LiftCnt_Ad : Sum
  MCU0_LiftCnt_Convert : DataTypeConversion  OutDataTypeStr=uint32
  MCU0_LiftCnt_F : Gain
  MCU0_LiftCnt_L : simulink/Logic and Bit Operations/Bitwise Operator  logicop=AND  UseBitMask=on  BitMask=255  BitMaskRealWorld=Stored Integer
  MCU0_LiftCnt_O : Constant  Value=0  OutDataTypeStr=single
  MCU0_LiftCnt_S : ArithShift
  MCU0_LiftCnt_Sub : Subsystem
  MCU0_LiftCnt_sat : Saturate  UpperLimit=255  LowerLimit=0
  MCU0_LiftCntcv : DataTypeConversion
  MCU0_ShutDowAllow_Ad : Sum
  MCU0_ShutDowAllow_Convert : DataTypeConversion  OutDataTypeStr=uint32
  MCU0_ShutDowAllow_F : Gain
  MCU0_ShutDowAllow_L : simulink/Logic and Bit Operations/Bitwise Operator  logicop=AND  UseBitMask=on  BitMask=64  BitMaskRealWorld=Stored Integer
  MCU0_ShutDowAllow_O : Constant  Value=0  OutDataTypeStr=single
  MCU0_ShutDowAllow_S : ArithShift  BitShiftNumber=6
  MCU0_ShutDowAllow_Sub : Subsystem
  MCU0_ShutDowAllow_sat : Saturate  UpperLimit=1  LowerLimit=0
  MCU0_ShutDowAllowcv : DataTypeConversion
  MCU0_SpeedFdk_Ad : Sum
  MCU0_SpeedFdk_Convert : DataTypeConversion  OutDataTypeStr=uint32
  MCU0_SpeedFdk_F : Gain
  MCU0_SpeedFdk_L : simulink/Logic and Bit Operations/Bitwise Operator  logicop=AND  UseBitMask=on  BitMask=65535  BitMaskRealWorld=Stored Integer
  MCU0_SpeedFdk_O : Constant  Value=-10000  OutDataTypeStr=single
  MCU0_SpeedFdk_S : ArithShift
  MCU0_SpeedFdk_Sub : Subsystem
  MCU0_SpeedFdk_sat : Saturate  UpperLimit=10000  LowerLimit=-10000
  MCU0_SpeedFdkcv : DataTypeConversion
  MCU0_SpeedFdkinput2_Ad : Sum
  MCU0_SpeedFdkinput2_C : Constant  Value=256
  MCU0_SpeedFdkinput2_P : Product
  MCU0_TorqueFdk_Ad : Sum
  MCU0_TorqueFdk_Convert : DataTypeConversion  OutDataTypeStr=uint32
  MCU0_TorqueFdk_F : Gain  Gain=0.1
  MCU0_TorqueFdk_L : simulink/Logic and Bit Operations/Bitwise Operator  logicop=AND  UseBitMask=on  BitMask=65535  BitMaskRealWorld=Stored Integer
  MCU0_TorqueFdk_O : Constant  Value=-1000  OutDataTypeStr=single
  MCU0_TorqueFdk_S : ArithShift
  MCU0_TorqueFdk_Sub : Subsystem
  MCU0_TorqueFdk_sat : Saturate  UpperLimit=1000  LowerLimit=-1000
  MCU0_TorqueFdkcv : DataTypeConversion
  MCU0_TorqueFdkinput4_Ad : Sum
  MCU0_TorqueFdkinput4_C : Constant  Value=256
  MCU0_TorqueFdkinput4_P : Product
  MCU0_TorqueMax_Ad : Sum
  MCU0_TorqueMax_Convert : DataTypeConversion  OutDataTypeStr=uint32
  MCU0_TorqueMax_F : Gain  Gain=0.1
  MCU0_TorqueMax_L : simulink/Logic and Bit Operations/Bitwise Operator  logicop=AND  UseBitMask=on  BitMask=65535  BitMaskRealWorld=Stored Integer
  MCU0_TorqueMax_O : Constant  Value=-1000  OutDataTypeStr=single
  MCU0_TorqueMax_S : ArithShift
  MCU0_TorqueMax_Sub : Subsystem
  MCU0_TorqueMax_sat : Saturate  UpperLimit=1000  LowerLimit=-1000
  MCU0_TorqueMaxcv : DataTypeConversion
  MCU0_TorqueMaxinput6_Ad : Sum
  MCU0_TorqueMaxinput6_C : Constant  Value=256
  MCU0_TorqueMaxinput6_P : Product
  MCU0_WorkStatus_Ad : Sum
  MCU0_WorkStatus_Convert : DataTypeConversion  OutDataTypeStr=uint32
  MCU0_WorkStatus_F : Gain
  MCU0_WorkStatus_L : simulink/Logic and Bit Operations/Bitwise Operator  logicop=AND  UseBitMask=on  BitMask=3  BitMaskRealWorld=Stored Integer
  MCU0_WorkStatus_O : Constant  Value=0  OutDataTypeStr=single
  MCU0_WorkStatus_S : ArithShift
  MCU0_WorkStatus_Sub : Subsystem
  MCU0_WorkStatus_sat : Saturate  UpperLimit=3  LowerLimit=0
  MCU0_WorkStatuscv : DataTypeConversion
  MCU0_TorqueMax_Out : Outport
  MCU0_EmergShutDown_Out : Outport  Port=2
  MCU0_ShutDowAllow_Out : Outport  Port=3
  MCU0_HighVol_Out : Outport  Port=4
  MCU0_LiftCnt_Out : Outport  Port=5
  MCU0_TorqueFdk_Out : Outport  Port=6
  MCU0_SpeedFdk_Out : Outport  Port=7
  MCU0_GearStatus_Out : Outport  Port=8
  MCU0_ControlMode_Out : Outport  Port=9
  MCU0_WorkStatus_Out : Outport  Port=10
  wires:
  MCU0_TorqueMax_F/1 -> MCU0_TorqueMax_Ad/1
  MCU0_TorqueMax_O/1 -> MCU0_TorqueMax_Ad/2
  MCU0_TorqueMax_Ad/1 -> MCU0_TorqueMax_sat/1
  MCU0_TorqueMax_sat/1 -> MCU0_TorqueMax_Out/1
  Demux/6 -> MCU0_TorqueMaxinput6_P/1
  MCU0_TorqueMaxinput6_C/1 -> MCU0_TorqueMaxinput6_P/2
  MCU0_TorqueMaxinput6_P/1 -> MCU0_TorqueMaxinput6_Ad/1
  Demux/7 -> MCU0_TorqueMaxinput6_Ad/2
  MCU0_TorqueMaxinput6_Ad/1 -> MCU0_TorqueMax_Sub/1(In1)
  MCU0_TorqueMax_Sub/1(Out1) -> MCU0_TorqueMax_Convert/1
  MCU0_TorqueMax_Convert/1 -> MCU0_TorqueMax_L/1
  MCU0_TorqueMax_L/1 -> MCU0_TorqueMax_S/1
  MCU0_TorqueMax_S/1 -> MCU0_TorqueMaxcv/1
  MCU0_TorqueMaxcv/1 -> MCU0_TorqueMax_F/1
  MCU0_EmergShutDown_F/1 -> MCU0_EmergShutDown_Ad/1
  MCU0_EmergShutDown_O/1 -> MCU0_EmergShutDown_Ad/2
  MCU0_EmergShutDown_Ad/1 -> MCU0_EmergShutDown_sat/1
  MCU0_EmergShutDown_sat/1 -> MCU0_EmergShutDown_Out/1
  Demux/1 -> MCU0_ControlMode_Sub/1(In1), MCU0_WorkStatus_Sub/1(In1), MCU0_GearStatus_Sub/1(In1), MCU0_HighVol_Sub/1(In1), MCU0_ShutDowAllow_Sub/1(In1), MCU0_EmergShutDown_Sub/1(In1)
  MCU0_EmergShutDown_Sub/1(Out1) -> MCU0_EmergShutDown_Convert/1
  MCU0_EmergShutDown_Convert/1 -> MCU0_EmergShutDown_L/1
  MCU0_EmergShutDown_L/1 -> MCU0_EmergShutDown_S/1
  MCU0_EmergShutDown_S/1 -> MCU0_EmergShutDowncv/1
  MCU0_EmergShutDowncv/1 -> MCU0_EmergShutDown_F/1
  MCU0_ShutDowAllow_F/1 -> MCU0_ShutDowAllow_Ad/1
  MCU0_ShutDowAllow_O/1 -> MCU0_ShutDowAllow_Ad/2
  MCU0_ShutDowAllow_Ad/1 -> MCU0_ShutDowAllow_sat/1
  MCU0_ShutDowAllow_sat/1 -> MCU0_ShutDowAllow_Out/1
  MCU0_ShutDowAllow_Sub/1(Out1) -> MCU0_ShutDowAllow_Convert/1
  MCU0_ShutDowAllow_Convert/1 -> MCU0_ShutDowAllow_L/1
  MCU0_ShutDowAllow_L/1 -> MCU0_ShutDowAllow_S/1
  MCU0_ShutDowAllow_S/1 -> MCU0_ShutDowAllowcv/1
  MCU0_ShutDowAllowcv/1 -> MCU0_ShutDowAllow_F/1
  MCU0_HighVol_F/1 -> MCU0_HighVol_Ad/1
  MCU0_HighVol_O/1 -> MCU0_HighVol_Ad/2
  MCU0_HighVol_Ad/1 -> MCU0_HighVol_sat/1
  MCU0_HighVol_sat/1 -> MCU0_HighVol_Out/1
  MCU0_HighVol_Sub/1(Out1) -> MCU0_HighVol_Convert/1
  MCU0_HighVol_Convert/1 -> MCU0_HighVol_L/1
  MCU0_HighVol_L/1 -> MCU0_HighVol_S/1
  MCU0_HighVol_S/1 -> MCU0_HighVolcv/1
  MCU0_HighVolcv/1 -> MCU0_HighVol_F/1
  MCU0_LiftCnt_F/1 -> MCU0_LiftCnt_Ad/1
  MCU0_LiftCnt_O/1 -> MCU0_LiftCnt_Ad/2
  MCU0_LiftCnt_Ad/1 -> MCU0_LiftCnt_sat/1
  MCU0_LiftCnt_sat/1 -> MCU0_LiftCnt_Out/1
  Demux/8 -> MCU0_LiftCnt_Sub/1(In1)
  MCU0_LiftCnt_Sub/1(Out1) -> MCU0_LiftCnt_Convert/1
  MCU0_LiftCnt_Convert/1 -> MCU0_LiftCnt_L/1
  MCU0_LiftCnt_L/1 -> MCU0_LiftCnt_S/1
  MCU0_LiftCnt_S/1 -> MCU0_LiftCntcv/1
  MCU0_LiftCntcv/1 -> MCU0_LiftCnt_F/1
  MCU0_TorqueFdk_F/1 -> MCU0_TorqueFdk_Ad/1
  MCU0_TorqueFdk_O/1 -> MCU0_TorqueFdk_Ad/2
  MCU0_TorqueFdk_Ad/1 -> MCU0_TorqueFdk_sat/1
  MCU0_TorqueFdk_sat/1 -> MCU0_TorqueFdk_Out/1
  Demux/4 -> MCU0_TorqueFdkinput4_P/1
  MCU0_TorqueFdkinput4_C/1 -> MCU0_TorqueFdkinput4_P/2
  MCU0_TorqueFdkinput4_P/1 -> MCU0_TorqueFdkinput4_Ad/1
  Demux/5 -> MCU0_TorqueFdkinput4_Ad/2
  MCU0_TorqueFdkinput4_Ad/1 -> MCU0_TorqueFdk_Sub/1(In1)
  MCU0_TorqueFdk_Sub/1(Out1) -> MCU0_TorqueFdk_Convert/1
  MCU0_TorqueFdk_Convert/1 -> MCU0_TorqueFdk_L/1
  MCU0_TorqueFdk_L/1 -> MCU0_TorqueFdk_S/1
  MCU0_TorqueFdk_S/1 -> MCU0_TorqueFdkcv/1
  MCU0_TorqueFdkcv/1 -> MCU0_TorqueFdk_F/1
  MCU0_SpeedFdk_F/1 -> MCU0_SpeedFdk_Ad/1
  MCU0_SpeedFdk_O/1 -> MCU0_SpeedFdk_Ad/2
  MCU0_SpeedFdk_Ad/1 -> MCU0_SpeedFdk_sat/1
  MCU0_SpeedFdk_sat/1 -> MCU0_SpeedFdk_Out/1
  Demux/2 -> MCU0_SpeedFdkinput2_P/1
  MCU0_SpeedFdkinput2_C/1 -> MCU0_SpeedFdkinput2_P/2
  MCU0_SpeedFdkinput2_P/1 -> MCU0_SpeedFdkinput2_Ad/1
  Demux/3 -> MCU0_SpeedFdkinput2_Ad/2
  MCU0_SpeedFdkinput2_Ad/1 -> MCU0_SpeedFdk_Sub/1(In1)
  MCU0_SpeedFdk_Sub/1(Out1) -> MCU0_SpeedFdk_Convert/1
  MCU0_SpeedFdk_Convert/1 -> MCU0_SpeedFdk_L/1
  MCU0_SpeedFdk_L/1 -> MCU0_SpeedFdk_S/1
  MCU0_SpeedFdk_S/1 -> MCU0_SpeedFdkcv/1
  MCU0_SpeedFdkcv/1 -> MCU0_SpeedFdk_F/1
  MCU0_GearStatus_F/1 -> MCU0_GearStatus_Ad/1
  MCU0_GearStatus_O/1 -> MCU0_GearStatus_Ad/2
  MCU0_GearStatus_Ad/1 -> MCU0_GearStatus_sat/1
  MCU0_GearStatus_sat/1 -> MCU0_GearStatus_Out/1
  MCU0_GearStatus_Sub/1(Out1) -> MCU0_GearStatus_Convert/1
  MCU0_GearStatus_Convert/1 -> MCU0_GearStatus_L/1
  MCU0_GearStatus_L/1 -> MCU0_GearStatus_S/1
  MCU0_GearStatus_S/1 -> MCU0_GearStatuscv/1
  MCU0_GearStatuscv/1 -> MCU0_GearStatus_F/1
  MCU0_ControlMode_F/1 -> MCU0_ControlMode_Ad/1
  MCU0_ControlMode_O/1 -> MCU0_ControlMode_Ad/2
  MCU0_ControlMode_Ad/1 -> MCU0_ControlMode_sat/1
  MCU0_ControlMode_sat/1 -> MCU0_ControlMode_Out/1
  MCU0_ControlMode_Sub/1(Out1) -> MCU0_ControlMode_Convert/1
  MCU0_ControlMode_Convert/1 -> MCU0_ControlMode_L/1
  MCU0_ControlMode_L/1 -> MCU0_ControlMode_S/1
  MCU0_ControlMode_S/1 -> MCU0_ControlModecv/1
  MCU0_ControlModecv/1 -> MCU0_ControlMode_F/1
  MCU0_WorkStatus_F/1 -> MCU0_WorkStatus_Ad/1
  MCU0_WorkStatus_O/1 -> MCU0_WorkStatus_Ad/2
  MCU0_WorkStatus_Ad/1 -> MCU0_WorkStatus_sat/1
  MCU0_WorkStatus_sat/1 -> MCU0_WorkStatus_Out/1
  MCU0_WorkStatus_Sub/1(Out1) -> MCU0_WorkStatus_Convert/1
  MCU0_WorkStatus_Convert/1 -> MCU0_WorkStatus_L/1
  MCU0_WorkStatus_L/1 -> MCU0_WorkStatus_S/1
  MCU0_WorkStatus_S/1 -> MCU0_WorkStatuscv/1
  MCU0_WorkStatuscv/1 -> MCU0_WorkStatus_F/1
  input/1 -> Demux/1

== system six_plus_six_AcmsteeringV09_main_2lflm/Data_input/MCU0_4/MCU0 ==
  input : Inport
  Enable : EnablePort
  Demux : Demux  Outputs=8
  MCU0_ControlMode_Ad : Sum
  MCU0_ControlMode_Convert : DataTypeConversion  OutDataTypeStr=uint32
  MCU0_ControlMode_F : Gain
  MCU0_ControlMode_L : simulink/Logic and Bit Operations/Bitwise Operator  logicop=AND  UseBitMask=on  BitMask=4  BitMaskRealWorld=Stored Integer
  MCU0_ControlMode_O : Constant  Value=0  OutDataTypeStr=single
  MCU0_ControlMode_S : ArithShift  BitShiftNumber=2
  MCU0_ControlMode_Sub : Subsystem
  MCU0_ControlMode_sat : Saturate  UpperLimit=1  LowerLimit=0
  MCU0_ControlModecv : DataTypeConversion
  MCU0_EmergShutDown_Ad : Sum
  MCU0_EmergShutDown_Convert : DataTypeConversion  OutDataTypeStr=uint32
  MCU0_EmergShutDown_F : Gain
  MCU0_EmergShutDown_L : simulink/Logic and Bit Operations/Bitwise Operator  logicop=AND  UseBitMask=on  BitMask=128  BitMaskRealWorld=Stored Integer
  MCU0_EmergShutDown_O : Constant  Value=0  OutDataTypeStr=single
  MCU0_EmergShutDown_S : ArithShift  BitShiftNumber=7
  MCU0_EmergShutDown_Sub : Subsystem
  MCU0_EmergShutDown_sat : Saturate  UpperLimit=1  LowerLimit=0
  MCU0_EmergShutDowncv : DataTypeConversion
  MCU0_GearStatus_Ad : Sum
  MCU0_GearStatus_Convert : DataTypeConversion  OutDataTypeStr=uint32
  MCU0_GearStatus_F : Gain
  MCU0_GearStatus_L : simulink/Logic and Bit Operations/Bitwise Operator  logicop=AND  UseBitMask=on  BitMask=24  BitMaskRealWorld=Stored Integer
  MCU0_GearStatus_O : Constant  Value=0  OutDataTypeStr=single
  MCU0_GearStatus_S : ArithShift  BitShiftNumber=3
  MCU0_GearStatus_Sub : Subsystem
  MCU0_GearStatus_sat : Saturate  UpperLimit=3  LowerLimit=0
  MCU0_GearStatuscv : DataTypeConversion
  MCU0_HighVol_Ad : Sum
  MCU0_HighVol_Convert : DataTypeConversion  OutDataTypeStr=uint32
  MCU0_HighVol_F : Gain
  MCU0_HighVol_L : simulink/Logic and Bit Operations/Bitwise Operator  logicop=AND  UseBitMask=on  BitMask=32  BitMaskRealWorld=Stored Integer
  MCU0_HighVol_O : Constant  Value=0  OutDataTypeStr=single
  MCU0_HighVol_S : ArithShift  BitShiftNumber=5
  MCU0_HighVol_Sub : Subsystem
  MCU0_HighVol_sat : Saturate  UpperLimit=1  LowerLimit=0
  MCU0_HighVolcv : DataTypeConversion
  MCU0_LiftCnt_Ad : Sum
  MCU0_LiftCnt_Convert : DataTypeConversion  OutDataTypeStr=uint32
  MCU0_LiftCnt_F : Gain
  MCU0_LiftCnt_L : simulink/Logic and Bit Operations/Bitwise Operator  logicop=AND  UseBitMask=on  BitMask=255  BitMaskRealWorld=Stored Integer
  MCU0_LiftCnt_O : Constant  Value=0  OutDataTypeStr=single
  MCU0_LiftCnt_S : ArithShift
  MCU0_LiftCnt_Sub : Subsystem
  MCU0_LiftCnt_sat : Saturate  UpperLimit=255  LowerLimit=0
  MCU0_LiftCntcv : DataTypeConversion
  MCU0_ShutDowAllow_Ad : Sum
  MCU0_ShutDowAllow_Convert : DataTypeConversion  OutDataTypeStr=uint32
  MCU0_ShutDowAllow_F : Gain
  MCU0_ShutDowAllow_L : simulink/Logic and Bit Operations/Bitwise Operator  logicop=AND  UseBitMask=on  BitMask=64  BitMaskRealWorld=Stored Integer
  MCU0_ShutDowAllow_O : Constant  Value=0  OutDataTypeStr=single
  MCU0_ShutDowAllow_S : ArithShift  BitShiftNumber=6
  MCU0_ShutDowAllow_Sub : Subsystem
  MCU0_ShutDowAllow_sat : Saturate  UpperLimit=1  LowerLimit=0
  MCU0_ShutDowAllowcv : DataTypeConversion
  MCU0_SpeedFdk_Ad : Sum
  MCU0_SpeedFdk_Convert : DataTypeConversion  OutDataTypeStr=uint32
  MCU0_SpeedFdk_F : Gain
  MCU0_SpeedFdk_L : simulink/Logic and Bit Operations/Bitwise Operator  logicop=AND  UseBitMask=on  BitMask=65535  BitMaskRealWorld=Stored Integer
  MCU0_SpeedFdk_O : Constant  Value=-10000  OutDataTypeStr=single
  MCU0_SpeedFdk_S : ArithShift
  MCU0_SpeedFdk_Sub : Subsystem
  MCU0_SpeedFdk_sat : Saturate  UpperLimit=10000  LowerLimit=-10000
  MCU0_SpeedFdkcv : DataTypeConversion
  MCU0_SpeedFdkinput2_Ad : Sum
  MCU0_SpeedFdkinput2_C : Constant  Value=256
  MCU0_SpeedFdkinput2_P : Product
  MCU0_TorqueFdk_Ad : Sum
  MCU0_TorqueFdk_Convert : DataTypeConversion  OutDataTypeStr=uint32
  MCU0_TorqueFdk_F : Gain  Gain=0.1
  MCU0_TorqueFdk_L : simulink/Logic and Bit Operations/Bitwise Operator  logicop=AND  UseBitMask=on  BitMask=65535  BitMaskRealWorld=Stored Integer
  MCU0_TorqueFdk_O : Constant  Value=-1000  OutDataTypeStr=single
  MCU0_TorqueFdk_S : ArithShift
  MCU0_TorqueFdk_Sub : Subsystem
  MCU0_TorqueFdk_sat : Saturate  UpperLimit=1000  LowerLimit=-1000
  MCU0_TorqueFdkcv : DataTypeConversion
  MCU0_TorqueFdkinput4_Ad : Sum
  MCU0_TorqueFdkinput4_C : Constant  Value=256
  MCU0_TorqueFdkinput4_P : Product
  MCU0_TorqueMax_Ad : Sum
  MCU0_TorqueMax_Convert : DataTypeConversion  OutDataTypeStr=uint32
  MCU0_TorqueMax_F : Gain  Gain=0.1
  MCU0_TorqueMax_L : simulink/Logic and Bit Operations/Bitwise Operator  logicop=AND  UseBitMask=on  BitMask=65535  BitMaskRealWorld=Stored Integer
  MCU0_TorqueMax_O : Constant  Value=-1000  OutDataTypeStr=single
  MCU0_TorqueMax_S : ArithShift
  MCU0_TorqueMax_Sub : Subsystem
  MCU0_TorqueMax_sat : Saturate  UpperLimit=1000  LowerLimit=-1000
  MCU0_TorqueMaxcv : DataTypeConversion
  MCU0_TorqueMaxinput6_Ad : Sum
  MCU0_TorqueMaxinput6_C : Constant  Value=256
  MCU0_TorqueMaxinput6_P : Product
  MCU0_WorkStatus_Ad : Sum
  MCU0_WorkStatus_Convert : DataTypeConversion  OutDataTypeStr=uint32
  MCU0_WorkStatus_F : Gain
  MCU0_WorkStatus_L : simulink/Logic and Bit Operations/Bitwise Operator  logicop=AND  UseBitMask=on  BitMask=3  BitMaskRealWorld=Stored Integer
  MCU0_WorkStatus_O : Constant  Value=0  OutDataTypeStr=single
  MCU0_WorkStatus_S : ArithShift
  MCU0_WorkStatus_Sub : Subsystem
  MCU0_WorkStatus_sat : Saturate  UpperLimit=3  LowerLimit=0
  MCU0_WorkStatuscv : DataTypeConversion
  MCU0_TorqueMax_Out : Outport
  MCU0_EmergShutDown_Out : Outport  Port=2
  MCU0_ShutDowAllow_Out : Outport  Port=3
  MCU0_HighVol_Out : Outport  Port=4
  MCU0_LiftCnt_Out : Outport  Port=5
  MCU0_TorqueFdk_Out : Outport  Port=6
  MCU0_SpeedFdk_Out : Outport  Port=7
  MCU0_GearStatus_Out : Outport  Port=8
  MCU0_ControlMode_Out : Outport  Port=9
  MCU0_WorkStatus_Out : Outport  Port=10
  wires:
  MCU0_TorqueMax_F/1 -> MCU0_TorqueMax_Ad/1
  MCU0_TorqueMax_O/1 -> MCU0_TorqueMax_Ad/2
  MCU0_TorqueMax_Ad/1 -> MCU0_TorqueMax_sat/1
  MCU0_TorqueMax_sat/1 -> MCU0_TorqueMax_Out/1
  Demux/6 -> MCU0_TorqueMaxinput6_P/1
  MCU0_TorqueMaxinput6_C/1 -> MCU0_TorqueMaxinput6_P/2
  MCU0_TorqueMaxinput6_P/1 -> MCU0_TorqueMaxinput6_Ad/1
  Demux/7 -> MCU0_TorqueMaxinput6_Ad/2
  MCU0_TorqueMaxinput6_Ad/1 -> MCU0_TorqueMax_Sub/1(In1)
  MCU0_TorqueMax_Sub/1(Out1) -> MCU0_TorqueMax_Convert/1
  MCU0_TorqueMax_Convert/1 -> MCU0_TorqueMax_L/1
  MCU0_TorqueMax_L/1 -> MCU0_TorqueMax_S/1
  MCU0_TorqueMax_S/1 -> MCU0_TorqueMaxcv/1
  MCU0_TorqueMaxcv/1 -> MCU0_TorqueMax_F/1
  MCU0_EmergShutDown_F/1 -> MCU0_EmergShutDown_Ad/1
  MCU0_EmergShutDown_O/1 -> MCU0_EmergShutDown_Ad/2
  MCU0_EmergShutDown_Ad/1 -> MCU0_EmergShutDown_sat/1
  MCU0_EmergShutDown_sat/1 -> MCU0_EmergShutDown_Out/1
  Demux/1 -> MCU0_ControlMode_Sub/1(In1), MCU0_WorkStatus_Sub/1(In1), MCU0_GearStatus_Sub/1(In1), MCU0_HighVol_Sub/1(In1), MCU0_ShutDowAllow_Sub/1(In1), MCU0_EmergShutDown_Sub/1(In1)
  MCU0_EmergShutDown_Sub/1(Out1) -> MCU0_EmergShutDown_Convert/1
  MCU0_EmergShutDown_Convert/1 -> MCU0_EmergShutDown_L/1
  MCU0_EmergShutDown_L/1 -> MCU0_EmergShutDown_S/1
  MCU0_EmergShutDown_S/1 -> MCU0_EmergShutDowncv/1
  MCU0_EmergShutDowncv/1 -> MCU0_EmergShutDown_F/1
  MCU0_ShutDowAllow_F/1 -> MCU0_ShutDowAllow_Ad/1
  MCU0_ShutDowAllow_O/1 -> MCU0_ShutDowAllow_Ad/2
  MCU0_ShutDowAllow_Ad/1 -> MCU0_ShutDowAllow_sat/1
  MCU0_ShutDowAllow_sat/1 -> MCU0_ShutDowAllow_Out/1
  MCU0_ShutDowAllow_Sub/1(Out1) -> MCU0_ShutDowAllow_Convert/1
  MCU0_ShutDowAllow_Convert/1 -> MCU0_ShutDowAllow_L/1
  MCU0_ShutDowAllow_L/1 -> MCU0_ShutDowAllow_S/1
  MCU0_ShutDowAllow_S/1 -> MCU0_ShutDowAllowcv/1
  MCU0_ShutDowAllowcv/1 -> MCU0_ShutDowAllow_F/1
  MCU0_HighVol_F/1 -> MCU0_HighVol_Ad/1
  MCU0_HighVol_O/1 -> MCU0_HighVol_Ad/2
  MCU0_HighVol_Ad/1 -> MCU0_HighVol_sat/1
  MCU0_HighVol_sat/1 -> MCU0_HighVol_Out/1
  MCU0_HighVol_Sub/1(Out1) -> MCU0_HighVol_Convert/1
  MCU0_HighVol_Convert/1 -> MCU0_HighVol_L/1
  MCU0_HighVol_L/1 -> MCU0_HighVol_S/1
  MCU0_HighVol_S/1 -> MCU0_HighVolcv/1
  MCU0_HighVolcv/1 -> MCU0_HighVol_F/1
  MCU0_LiftCnt_F/1 -> MCU0_LiftCnt_Ad/1
  MCU0_LiftCnt_O/1 -> MCU0_LiftCnt_Ad/2
  MCU0_LiftCnt_Ad/1 -> MCU0_LiftCnt_sat/1
  MCU0_LiftCnt_sat/1 -> MCU0_LiftCnt_Out/1
  Demux/8 -> MCU0_LiftCnt_Sub/1(In1)
  MCU0_LiftCnt_Sub/1(Out1) -> MCU0_LiftCnt_Convert/1
  MCU0_LiftCnt_Convert/1 -> MCU0_LiftCnt_L/1
  MCU0_LiftCnt_L/1 -> MCU0_LiftCnt_S/1
  MCU0_LiftCnt_S/1 -> MCU0_LiftCntcv/1
  MCU0_LiftCntcv/1 -> MCU0_LiftCnt_F/1
  MCU0_TorqueFdk_F/1 -> MCU0_TorqueFdk_Ad/1
  MCU0_TorqueFdk_O/1 -> MCU0_TorqueFdk_Ad/2
  MCU0_TorqueFdk_Ad/1 -> MCU0_TorqueFdk_sat/1
  MCU0_TorqueFdk_sat/1 -> MCU0_TorqueFdk_Out/1
  Demux/4 -> MCU0_TorqueFdkinput4_P/1
  MCU0_TorqueFdkinput4_C/1 -> MCU0_TorqueFdkinput4_P/2
  MCU0_TorqueFdkinput4_P/1 -> MCU0_TorqueFdkinput4_Ad/1
  Demux/5 -> MCU0_TorqueFdkinput4_Ad/2
  MCU0_TorqueFdkinput4_Ad/1 -> MCU0_TorqueFdk_Sub/1(In1)
  MCU0_TorqueFdk_Sub/1(Out1) -> MCU0_TorqueFdk_Convert/1
  MCU0_TorqueFdk_Convert/1 -> MCU0_TorqueFdk_L/1
  MCU0_TorqueFdk_L/1 -> MCU0_TorqueFdk_S/1
  MCU0_TorqueFdk_S/1 -> MCU0_TorqueFdkcv/1
  MCU0_TorqueFdkcv/1 -> MCU0_TorqueFdk_F/1
  MCU0_SpeedFdk_F/1 -> MCU0_SpeedFdk_Ad/1
  MCU0_SpeedFdk_O/1 -> MCU0_SpeedFdk_Ad/2
  MCU0_SpeedFdk_Ad/1 -> MCU0_SpeedFdk_sat/1
  MCU0_SpeedFdk_sat/1 -> MCU0_SpeedFdk_Out/1
  Demux/2 -> MCU0_SpeedFdkinput2_P/1
  MCU0_SpeedFdkinput2_C/1 -> MCU0_SpeedFdkinput2_P/2
  MCU0_SpeedFdkinput2_P/1 -> MCU0_SpeedFdkinput2_Ad/1
  Demux/3 -> MCU0_SpeedFdkinput2_Ad/2
  MCU0_SpeedFdkinput2_Ad/1 -> MCU0_SpeedFdk_Sub/1(In1)
  MCU0_SpeedFdk_Sub/1(Out1) -> MCU0_SpeedFdk_Convert/1
  MCU0_SpeedFdk_Convert/1 -> MCU0_SpeedFdk_L/1
  MCU0_SpeedFdk_L/1 -> MCU0_SpeedFdk_S/1
  MCU0_SpeedFdk_S/1 -> MCU0_SpeedFdkcv/1
  MCU0_SpeedFdkcv/1 -> MCU0_SpeedFdk_F/1
  MCU0_GearStatus_F/1 -> MCU0_GearStatus_Ad/1
  MCU0_GearStatus_O/1 -> MCU0_GearStatus_Ad/2
  MCU0_GearStatus_Ad/1 -> MCU0_GearStatus_sat/1
  MCU0_GearStatus_sat/1 -> MCU0_GearStatus_Out/1
  MCU0_GearStatus_Sub/1(Out1) -> MCU0_GearStatus_Convert/1
  MCU0_GearStatus_Convert/1 -> MCU0_GearStatus_L/1
  MCU0_GearStatus_L/1 -> MCU0_GearStatus_S/1
  MCU0_GearStatus_S/1 -> MCU0_GearStatuscv/1
  MCU0_GearStatuscv/1 -> MCU0_GearStatus_F/1
  MCU0_ControlMode_F/1 -> MCU0_ControlMode_Ad/1
  MCU0_ControlMode_O/1 -> MCU0_ControlMode_Ad/2
  MCU0_ControlMode_Ad/1 -> MCU0_ControlMode_sat/1
  MCU0_ControlMode_sat/1 -> MCU0_ControlMode_Out/1
  MCU0_ControlMode_Sub/1(Out1) -> MCU0_ControlMode_Convert/1
  MCU0_ControlMode_Convert/1 -> MCU0_ControlMode_L/1
  MCU0_ControlMode_L/1 -> MCU0_ControlMode_S/1
  MCU0_ControlMode_S/1 -> MCU0_ControlModecv/1
  MCU0_ControlModecv/1 -> MCU0_ControlMode_F/1
  MCU0_WorkStatus_F/1 -> MCU0_WorkStatus_Ad/1
  MCU0_WorkStatus_O/1 -> MCU0_WorkStatus_Ad/2
  MCU0_WorkStatus_Ad/1 -> MCU0_WorkStatus_sat/1
  MCU0_WorkStatus_sat/1 -> MCU0_WorkStatus_Out/1
  MCU0_WorkStatus_Sub/1(Out1) -> MCU0_WorkStatus_Convert/1
  MCU0_WorkStatus_Convert/1 -> MCU0_WorkStatus_L/1
  MCU0_WorkStatus_L/1 -> MCU0_WorkStatus_S/1
  MCU0_WorkStatus_S/1 -> MCU0_WorkStatuscv/1
  MCU0_WorkStatuscv/1 -> MCU0_WorkStatus_F/1
  input/1 -> Demux/1

== matlab function six_plus_six_AcmsteeringV09_main_2lflm/MainControl/mode_control/backward/backward/Drive/目标转向力矩确定模块/MATLAB Function ==
  data: steer_dem input; Rturn_min output; G input; L input; umax input; B input; Tpeak_L input; Tpeak_R input; eff_tran input; Radius input; f input
function Rturn_min = fcn(steer_dem,G,L,umax,B,Tpeak_L,Tpeak_R,eff_tran,Radius,f)
%#codegen
if steer_dem>0
    Rturn_min=single((G*L*umax/(4*B*(Tpeak_R*eff_tran/Radius-f*G/2))-0.925)/0.15*B);
else
    Rturn_min=single((G*L*umax/(4*B*(Tpeak_L*eff_tran/Radius-f*G/2))-0.925)/0.15*B);
end
end

== matlab function six_plus_six_AcmsteeringV09_main_2lflm/MainControl/mode_control/backward/backward/Drive/驱动防滑控制TCS/直行TCS/直行/HeartBeat ==
  data: life_pre input; life output
function life = fcn(life_pre)
%#codegen
life=single(life_pre+1);
if life>255
    life=single(0);
end
end

== matlab function six_plus_six_AcmsteeringV09_main_2lflm/MainControl/mode_control/backward/backward/Drive/驱动防滑控制TCS/直行TCS/直行/HeartBeat2 ==
  data: life_pre input; life output
function life = fcn(life_pre)
%#codegen
life=single(life_pre+1);
if life>255
    life=single(0);
end
end

== matlab function six_plus_six_AcmsteeringV09_main_2lflm/MainControl/mode_control/backward/backward/Drive/驱动防滑控制TCS/直行TCS/直行/HeartBeat5 ==
  data: life_pre input; life output
function life = fcn(life_pre)
%#codegen
life=single(life_pre+1);
if life>255
    life=single(0);
end
end

== matlab function six_plus_six_AcmsteeringV09_main_2lflm/MainControl/mode_control/center_steer/center_steer/HeartBeat2 ==
  data: life_pre input; life output
function life = fcn(life_pre)
%#codegen
life=single(life_pre+1);
if life>255
    life=single(0);
end
end
